simulink model "GroundSourceHX_newGfunction"  (R2018b)
settings: Solver=ode23t  StartTime=0.0  StopTime=30*365*24*3600  RelTol=1e-3
libraries: carnot x6
settings Model: SimulationMode=accelerator  Creator=goettsche  LastModifiedBy=drhf
settings DataIOCC: SaveOutput=off  SignalLogging=off  DSMLogging=off  SaveTime=off
settings DebuggingCC: ReadBeforeWriteMsg=DisableAll  WriteAfterWriteMsg=DisableAll  WriteAfterReadMsg=DisableAll  MultiTaskDSMMsg=none
settings ModelReferenceCC: UpdateModelReferenceTargets=IfOutOfDate
settings SFSimCC: SFSimEcho=off

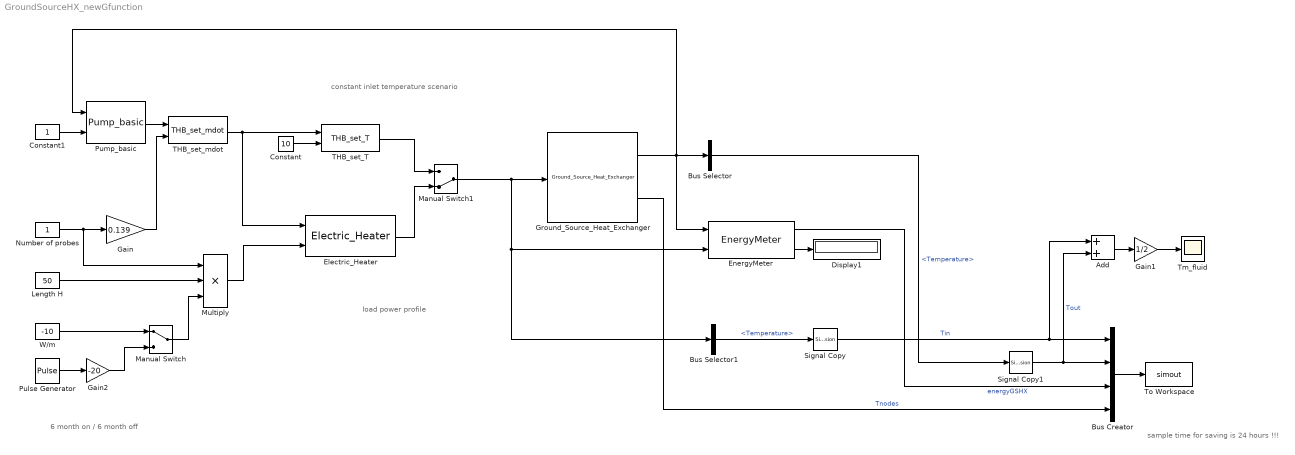
== system GroundSourceHX_newGfunction ==
  note: constant inlet temperature scenario
  note: sample time for saving is 24 hours !!!
  note: load power profile
  note: 6 month on / 6 month off
  Add : Sum
  Bus Creator : BusCreator  Inputs=4
  Bus Selector : BusSelector  OutputSignals=Temperature
  Bus Selector1 : BusSelector  OutputSignals=Temperature
  Constant : Constant  Value=10
  Constant1 : Constant
  Display1 : Display
  Electric_Heater : carnot/Source/Boiler/Electric_Heater
      settings: SourceProductName=Carnot
  EnergyMeter : carnot/Control/EnergyMeter
      settings: SourceProductName=Carnot
  Gain : Gain  Gain=0.139
  Gain1 : Gain  Gain=1/2
  Gain2 : Gain  Gain=-20
  Ground_Source_Heat_Exchanger : carnot/Source/Heat_Pump/Ground_Source_Heat_Exchanger  Jahresmitteltemp_C=0  TGrad=0  lambdaErde=2.5  cpErde=1000  rhoErde=2200  lambdaFill=0.81  cpFill=3040  rhoFill=1180  lambda_Sondenrohr=0.48  dTdesign=5  Sondenlaenge=100  B_sondenabstand=10  Sondendurchmesser=0.026+2*0.003  Bohrdurchmesser=0.12  Bu_param=0.06  Wanddicke_Sondenrohr=0.003  SondenFall=1 probe  DimVert=5  DimRad=10  Gitterfaktor=1.5  LastYear=1  show=on
      settings: SourceProductName=Carnot
  Length H : Constant  Value=50
  Manual Switch : ManualSwitch
  Manual Switch1 : ManualSwitch  CurrentSetting=0
  Multiply : Product  Inputs=3
  Number of probes : Constant
  Pulse Generator : DiscretePulseGenerator  PulseType=Time based  Period=3600*8760  PulseWidth=50
  Pump_basic : carnot/Hydraulics/Pump_basic  mdotmax=0.1  fluid_id=Water-Glycol Mix  mix=0.25  mix2=0  mix3=0  p0=1e5  dia=0.02  ID=No Pressure Drop  hgt=0
      settings: SourceProductName=Carnot
  Signal Copy : SignalConversion  OverrideOpt=off
  Signal Copy1 : SignalConversion  OverrideOpt=off
  THB_set_T : carnot/Source/Simple/THB_set_T
      settings: SourceProductName=Carnot
  THB_set_mdot : carnot/Source/Simple/THB_set_mdot
      settings: SourceProductName=Carnot
  Tm_fluid : Scope
  To Workspace : ToWorkspace  VariableName=simout  SaveFormat=Timeseries  SampleTime=24*3600
  W/m : Constant  Value=-10
  wires:
  Ground_Source_Heat_Exchanger/1 -> Pump_basic/1, Bus Selector/1, EnergyMeter/1
  Bus Selector/1 -> Signal Copy1/1  "<Temperature>"
  Manual Switch1/1 -> Ground_Source_Heat_Exchanger/1, EnergyMeter/2, Bus Selector1/1
  THB_set_mdot/1 -> THB_set_T/1, Electric_Heater/1
  Bus Selector1/1 -> Signal Copy/1  "<Temperature>"
  Ground_Source_Heat_Exchanger/2 -> Bus Creator/4  "Tnodes"
  Signal Copy/1 -> Add/1, Bus Creator/1  "Tin"
  Signal Copy1/1 -> Add/2, Bus Creator/2  "Tout"
  Bus Creator/1 -> To Workspace/1
  EnergyMeter/1 -> Bus Creator/3  "energyGSHX"
  EnergyMeter/2 -> Display1/1
  Gain/1 -> THB_set_mdot/2
  Number of probes/1 -> Multiply/1, Gain/1
  Multiply/1 -> Electric_Heater/2
  Pump_basic/1 -> THB_set_mdot/1
  Constant1/1 -> Pump_basic/2
  Length H/1 -> Multiply/2
  Add/1 -> Gain1/1
  Gain1/1 -> Tm_fluid/1
  Pulse Generator/1 -> Gain2/1
  W/m/1 -> Manual Switch/1
  Gain2/1 -> Manual Switch/2
  Electric_Heater/1 -> Manual Switch1/2
  THB_set_T/1 -> Manual Switch1/1
  Manual Switch/1 -> Multiply/3
  Constant/1 -> THB_set_T/2
